simulink model "ModelPrev"  (R2020a)
settings: Solver=VariableStepAuto  StartTime=0.0  StopTime=20  RelTol=1e-3
libraries: fl_lib x7, nesl_utility x6, SimscapeFluids_lib x4
settings Model: Creator=parthmahendru  LastModifiedBy=parthmahendru

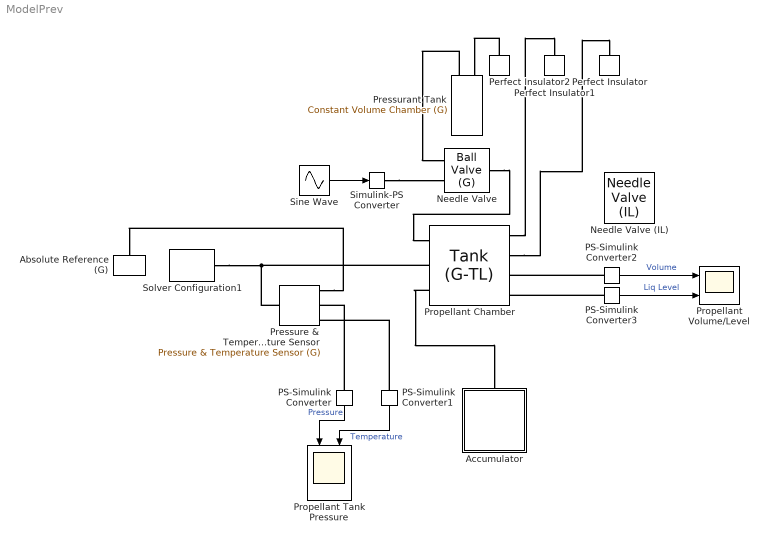
== system ModelPrev ==
  Absolute Reference (G) : fl_lib/Gas/Elements/Absolute Reference (G)
      settings: SourceProductBaseCode=SS  InternalSimscapePortConfiguration="{\"Bottom\":[],\"Left\":[{\"id\":\"A\",\"label\":\"\",\"type\":\"foundation.gas.gas\"}],\"Right\":[],\"Top\":[]}"
  Accumulator : Subsystem
  Needle Valve : SimscapeFluids_lib/Gas/Valves & Orifices/Flow Control Valves/Ball Valve (G)  valve_seat_spec=fluids.gas.enum.ball_valve_spec.sharp  cone_angle=120 deg  diam_ball=0.01 m  diam_orifice=7e-3 m  x0=0  iso_cond_spec=fluids.gas.enum.flow_control_valve_spec.Cv  C_max=1.6 l/s/bar  B_crit=0.3  m=0.5  Cv_max=0.5  Kv_max=0.3  area_leak=1e-12 m^2  area=0.01 m^2  smoothing_factor=0  B_lam=0.999  T0=293.15 K  rho0=1.185 kg/m^3
      settings: SourceProductBaseCode=SH  InternalSimscapePortConfiguration="{\"Bottom\":[],\"Left\":[{\"id\":\"A\",\"label\":\"A\",\"type\":\"foundation.gas.gas\"},{\"id\":\"L\",\"label\":\"L\",\"type\":\"input\"}],\"Right\":[{\"id\":\"B\",\"label\":\"B\",\"type\":\"foundation.gas.gas\"}],\"Top\":[]}"
  Needle Valve (IL) : SimscapeFluids_lib/Isothermal Liquid/Valves & Orifices/Flow Control Valves/Needle Valve (IL)  diam_orifice=5e-3 m  cone_angle=90 deg  S_min=0 m  area_leak=1e-10 m^2  area=inf m^2  Cd=0.64  Re_c=150  pressure_recovery=simscape.enum.onoff.off  mdot_A_specify=off  mdot_A_priority=None  mdot_A=0 kg/s  mdot_A_nominal_specify=off  mdot_A_nominal_unit=kg/s  mdot_A_nominal_value=1  mdot_B_specify=off  mdot_B_priority=None  mdot_B=0 kg/s  mdot_B_nominal_specify=off  mdot_B_nominal_unit=kg/s  mdot_B_nominal_value=1
      settings: SourceProductBaseCode=SH  InternalSimscapePortConfiguration="{\"Bottom\":[],\"Left\":[{\"id\":\"A\",\"label\":\"A\",\"type\":\"foundation.isothermal_liquid.isothermal_liquid\"},{\"id\":\"S\",\"label\":\"S\",\"type\":\"input\"}],\"Right\":[{\"id\":\"B\",\"label\":\"B\",\"type\":\"foundation.isothermal_liquid.isothermal_liquid\"}],\"Top\":[]}"
  PS-Simulink Converter{,1..3} (4 alike) : nesl_utility/PS-Simulink Converter  PhysicalDomain=network_engine_domain  SubClassName=ps_output  LeftPortType=input  RightPortType=output  PseudoPeriodic=off  Frequencies=[]  Unit=inherit  AffineConversion=off
  Perfect Insulator : fl_lib/Thermal/Thermal Elements/Perfect Insulator  T_specify=off  T_priority=None  T=0 K  T_nominal_specify=off  T_nominal_unit=K  T_nominal_value=1
  Perfect Insulator1 : fl_lib/Thermal/Thermal Elements/Perfect Insulator  T_specify=off  T_priority=None  T=0 K  T_nominal_specify=off  T_nominal_unit=K  T_nominal_value=1
  Perfect Insulator2 : fl_lib/Thermal/Thermal Elements/Perfect Insulator  T_specify=off  T_priority=None  T=0 K  T_nominal_specify=off  T_nominal_unit=K  T_nominal_value=1
  Pressurant Tank : fl_lib/Gas/Elements/Constant Volume Chamber (G)  volume=20 m^3  num_ports=foundation.enum.num_ports.one  area_A=0.1 m^2  area_B=0.01 m^2  area_C=0.01 m^2  area_D=0.01 m^2  p_I_specify=on  p_I_priority=High  p_I=50 bar  p_I_nominal_specify=off  p_I_nominal_unit=MPa  p_I_nominal_value=1  T_I_specify=on  T_I_priority=High  T_I=293.15 K  T_I_nominal_specify=off  T_I_nominal_unit=K  T_I_nominal_value=1  rho_chamber_specify=on  rho_chamber_priority=High  rho_chamber=1.2 kg/m^3  rho_chamber_nominal_specify=off  rho_chamber_nominal_unit=kg/m^3  rho_chamber_nominal_value=1
      settings: SourceProductBaseCode=SS  InternalSimscapePortConfiguration="{\"Bottom\":[],\"Left\":[{\"id\":\"A\",\"label\":\"A\",\"type\":\"foundation.gas.gas\"},{\"id\":\"H\",\"label\":\"H\",\"type\":\"foundation.thermal.thermal\"}],\"Right\":[],\"Top\":[]}"
  "Pressure & Temperature Sensor " : fl_lib/Gas/Sensors/Pressure & Temperature Sensor (G)
      settings: SourceProductBaseCode=SS  InternalSimscapePortConfiguration="{\"Bottom\":[],\"Left\":[{\"id\":\"A\",\"label\":\"A\",\"type\":\"foundation.gas.gas\"}],\"Right\":[{\"id\":\"B\",\"label\":\"B\",\"type\":\"foundation.gas.gas\"},{\"id\":\"P\",\"label\":\"P\",\"type\":\"output\"},{\"id\":\"T\",\"label\":\"T\",\"type\":\"output\"}],\"Top\":[]}"
  Propellant Chamber : SimscapeFluids_lib/Fluid Network Interfaces/Tanks & Accumulators/Tank (G-TL)  volume_total=50 l  volume_spec=1  tank_area=5 m^2  level_TLU=[0, 3, 5] m  volume_TLU=[0, 4, 6] m^3  inlet_height=0.00001 m  inlet_areas_A1B1=[.01, .01] m^2  area_A2=0.0000001 m^2  g=9.81 m/s^2  p_gas_tank_specify=on  p_gas_tank_priority=High  p_gas_tank=10 bar  p_gas_tank_nominal_specify=off  p_gas_tank_nominal_unit=MPa  p_gas_tank_nominal_value=1  T_gas_tank_specify=on  T_gas_tank_priority=High  T_gas_tank=293.15 K  T_gas_tank_nominal_specify=off  T_gas_tank_nominal_unit=K  T_gas_tank_nominal_value=1  rho_gas_tank_specify=on  rho_gas_tank_priority=None  rho_gas_tank=1.2 kg/m^3  rho_gas_tank_nominal_specify=off  rho_gas_tank_nominal_unit=kg/m^3  rho_gas_tank_nominal_value=1  T_liquid_tank_specify=on  T_liquid_tank_priority=High  T_liquid_tank=293.15 K  T_liquid_tank_nominal_specify=off  T_liquid_tank_nominal_unit=K  T_liquid_tank_nominal_value=1  level_specify=on  level_priority=High  level=10 m  level_nominal_specify=off  level_nominal_unit=m  level_nominal_value=1  volume_liquid_specify=on  volume_liquid_priority=High  volume_liquid=20 l  volume_liquid_nominal_specify=off  volume_liquid_nominal_unit=m^3  volume_liquid_nominal_value=1  mass_liquid_specify=off  mass_liquid_priority=None  mass_liquid=5e+3 kg  mass_liquid_nominal_specify=off  mass_liquid_nominal_unit=kg  mass_liquid_nominal_value=1  inlet_heights_A2B2=[.1, 0] m  inlet_areas_A2B2=[.01, .01] m^2  inlet_heights_A2B2C2=[.1, .05, 0] m  inlet_areas_A2B2C2=[.01, .01, .01] m^2
      settings: SourceProductBaseCode=SH  InternalSimscapePortConfiguration="{\"Bottom\":[],\"Left\":[{\"id\":\"A1\",\"label\":\"A1\",\"type\":\"foundation.gas.gas\"},{\"id\":\"B1\",\"label\":\"B1\",\"type\":\"foundation.gas.gas\"},{\"id\":\"A2\",\"label\":\"A2\",\"type\":\"foundation.thermal_liquid.thermal_liquid\"}],\"Right\":[{\"id\":\"H1\",\"label\":\"H1\",\"type\":\"foundation.thermal.thermal\"},{\"id\":\"H2\",\"label\":\"H2\",\"type\":\"foundation.thermal.thermal\"},{\"id\":\"V_out\",\"label\":\"V\",\"type\":\"output\"},{\"id\":\"L_out\",\"label\":\"L\",\"type\":\"output\"}],\"Top\":[]}"
  Propellant Tank Pressure : Scope  NumInputPorts=2
  Propellant Volume/Level : Scope  NumInputPorts=2
  Simulink-PS Converter : nesl_utility/Simulink-PS Converter  PhysicalDomain=network_engine_domain  SubClassName=ps_input  LeftPortType=input  RightPortType=output  PseudoPeriodic=off  Frequencies=[]  NoiseDistribution=none  NoiseParameters=[]  Unit=1  AffineConversion=off  FilteringAndDerivatives=provide  SimscapeFilterOrder=1  InputFilterTimeConstant=0.001  UdotUserProvided=0
  Sine Wave : Sin  SampleTime=0
  Solver Configuration1 : nesl_utility/Solver Configuration  PhysicalDomain=network_engine_domain  SubClassName=solver  LeftPortType=input  RightPortType=generic  Tones=[]  Harmonics=[]  SimulateNoise=off  Profile=off  UseLocalSampling=off  EnableSwitchedLinearOptims=on  FrequencyDomain=off  UseCCode=off  RelTol=0.001  AbsTol=1e-06  MinStep=1e-09  ToWorkspace=off  RevertToSquareIcSolve=off  NumHomotopyIterations=100  PhasorMode=off  PhasorModeNumHarmonics=1  DoDC=off  ResidualTolerance=1e-09  UseLocalSolver=off  LocalSolverChoice=NE_BACKWARD_EULER_ADVANCER  LocalSolverSampleTime=0.001  DoFixedCost=off  MaxNonlinIter=3  MaxModeIter=2  LinearAlgebra=auto  EquationFormulation=NE_TIME_EF  DelaysMemoryBudget=1024  AutomaticFiltering=on  FilteringTimeConstant=0.001  PartitionStorageMethod=AS_NEEDED  PartitionMemoryBudget=1024  PartitionMethod=ROBUST
  wires:
  PS-Simulink Converter/1 -> Propellant Tank Pressure/1  "Pressure"
  PS-Simulink Converter1/1 -> Propellant Tank Pressure/2  "Temperature"
  PS-Simulink Converter2/1 -> Propellant Volume/Level/1  "Volume"
  PS-Simulink Converter3/1 -> Propellant Volume/Level/2  "Liq Level"
  Sine Wave/1 -> Simulink-PS Converter/1
  connections:
  PS-Simulink Converter/LConn1 -- "Pressure & Temperature Sensor "/RConn2
  PS-Simulink Converter1/LConn1 -- "Pressure & Temperature Sensor "/RConn3
  Propellant Chamber/RConn2 -- Perfect Insulator/LConn1
  "Pressure & Temperature Sensor "/RConn1 -- Absolute Reference (G)/LConn1
  "Pressure & Temperature Sensor "/LConn1 -- Propellant Chamber/LConn2 -- Solver Configuration1/RConn1
  Pressurant Tank/LConn1 -- Needle Valve/LConn1
  Propellant Chamber/RConn1 -- Perfect Insulator1/LConn1
  Perfect Insulator2/LConn1 -- Pressurant Tank/LConn2
  PS-Simulink Converter2/LConn1 -- Propellant Chamber/RConn3
  PS-Simulink Converter3/LConn1 -- Propellant Chamber/RConn4
  Needle Valve/RConn1 -- Propellant Chamber/LConn1
  Simulink-PS Converter/RConn1 -- Needle Valve/LConn2
  Propellant Chamber/LConn3 -- Accumulator/RConn1

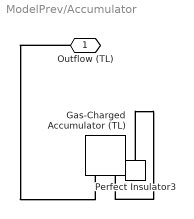
== system ModelPrev/Accumulator ==
  Gas-Charged Accumulator (TL) : SimscapeFluids_lib/Thermal Liquid/Tanks & Accumulators/Gas-Charged Accumulator (TL)  capacity=100 m^3  dead_volume=4e-5 m^3  p_precharge_gauge=0 MPa  k_sh=1.2  area=0.01 m^2  stiff_coeff=1e4 MPa/m^3  damping_coeff=1e4 s*MPa/m^6  liquid_volume_specify=off  liquid_volume_priority=High  liquid_volume=0.005 m^3  liquid_volume_nominal_specify=off  liquid_volume_nominal_unit=m^3  liquid_volume_nominal_value=1  liquid_mass_specify=off  liquid_mass_priority=None  liquid_mass=5 kg  liquid_mass_nominal_specify=off  liquid_mass_nominal_unit=kg  liquid_mass_nominal_value=1  p_accumulator_specify=off  p_accumulator_priority=None  p_accumulator=0.101325 MPa  p_accumulator_nominal_specify=off  p_accumulator_nominal_unit=MPa  p_accumulator_nominal_value=1  T_accumulator_specify=off  T_accumulator_priority=High  T_accumulator=293.15 K  T_accumulator_nominal_specify=off  T_accumulator_nominal_unit=K  T_accumulator_nominal_value=1
      settings: SourceProductBaseCode=SH  InternalSimscapePortConfiguration="{\"Bottom\":[],\"Left\":[],\"Right\":[{\"id\":\"A\",\"label\":\"A\",\"type\":\"foundation.thermal_liquid.thermal_liquid\"},{\"id\":\"H\",\"label\":\"H\",\"type\":\"foundation.thermal.thermal\"}],\"Top\":[]}"
  Perfect Insulator3 : fl_lib/Thermal/Thermal Elements/Perfect Insulator  T_specify=off  T_priority=None  T=0 K  T_nominal_specify=off  T_nominal_unit=K  T_nominal_value=1
  " Outflow (TL)" : PMIOPort  Side=Right
  connections:
  " Outflow (TL)"/RConn1 -- Gas-Charged Accumulator (TL)/RConn1
  Perfect Insulator3/LConn1 -- Gas-Charged Accumulator (TL)/RConn2
